simulink model "P_controller"  (R2019a)
settings: Solver=VariableStepAuto  StartTime=0.0  StopTime=2  RelTol=1e-3
values from neighbouring files (symbols this model uses):
  g = 9.81    [Data.m]    (also in func.m; myTransitionFcn.m)
  m = 0.1    [Data.m]    (also in myTransitionFcn.m)
  r = 0.1    [Data.m]    (also in func.m; myTransitionFcn.m)
  R = 1    [Data.m]    (also in func.m; myTransitionFcn.m)
libraries: simulink x1
settings Model: Creator=Dell  LastModifiedBy=Dell
settings SolverCC: AlgebraicLoopSolver=LineSearch

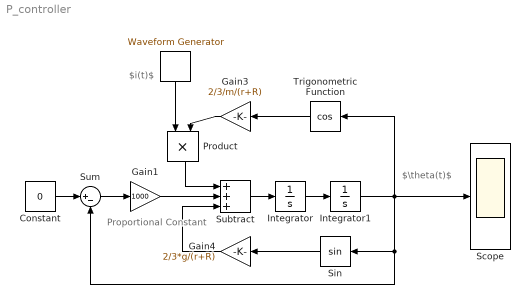
== system P_controller ==
  note: Proportional Constant
  note: $i(t)$
  note: $\theta(t)$
  " " : simulink/Sources/Waveform Generator  OutMin=[]  OutMax=[]  OutDataTypeStr=double  SelectedSignal=1  Signals=step(0,0,1)  BlockNames=MultiportSwitch_e98c01f307a14ef  SampleTime=0.1
      settings: SourceProductName=Simulink
  Constant : Constant  Value=0
  Gain1 : Gain  Gain=1000
  Gain3 : Gain  Gain=2/3/m/(r+R)
  Gain4 : Gain  Gain=2/3*g/(r+R)
  Integrator : Integrator
  Integrator1 : Integrator
  Product : Product
  Scope : Scope
  Sin : Trigonometry
  Subtract : Sum  Inputs=+++
  Sum : Sum  Inputs=|+-
  Trigonometric Function : Trigonometry  Operator=cos
  wires:
  Sum/1 -> Gain1/1
  Trigonometric Function/1 -> Gain3/1
  Constant/1 -> Sum/1
  Subtract/1 -> Integrator/1
  Product/1 -> Subtract/1
  Integrator1/1 -> Trigonometric Function/1, Scope/1, Sin/1, Sum/2
  Integrator/1 -> Integrator1/1
  Sin/1 -> Gain4/1
  Gain3/1 -> Product/2
  Gain4/1 -> Subtract/3
  Gain1/1 -> Subtract/2
  " "/1 -> Product/1
